simulink model "example_arduino_send_receive"  (R2015b)
settings: Solver=FixedStepAuto  StartTime=0.0  StopTime=1000  FixedStep=1/1000  RelTol=1e-3
libraries: SimFly_System x3
settings Model: ExtModeTrigDuration=2  Creator=marcell  LastModifiedBy=marcell
settings OptimizationCC: OptimizeModelRefInitCode=on  LifeSpan=1  MaxStackSize=64
settings HardwareCC: ProdBitPerPointer=32  ProdLargestAtomicInteger=Long  ProdLargestAtomicFloat=Double  ProdWordSize=32  ProdHWDeviceType=ARM Compatible->ARM Cortex
settings RTWCC: SystemTargetFile=ert.tlc  TemplateMakefile=ert_default_tmf  Description=Embedded Coder  CustomSource=arduino_DUE_wrapper.cpp  Toolchain=Arduino ARM v1.6.1  BuildConfiguration=Faster Runs
settings CodeAppCC: IgnoreCustomStorageClasses=off
settings ERTTargetCC: SupportContinuousTime=on  SupportVariableSizeSignals=on

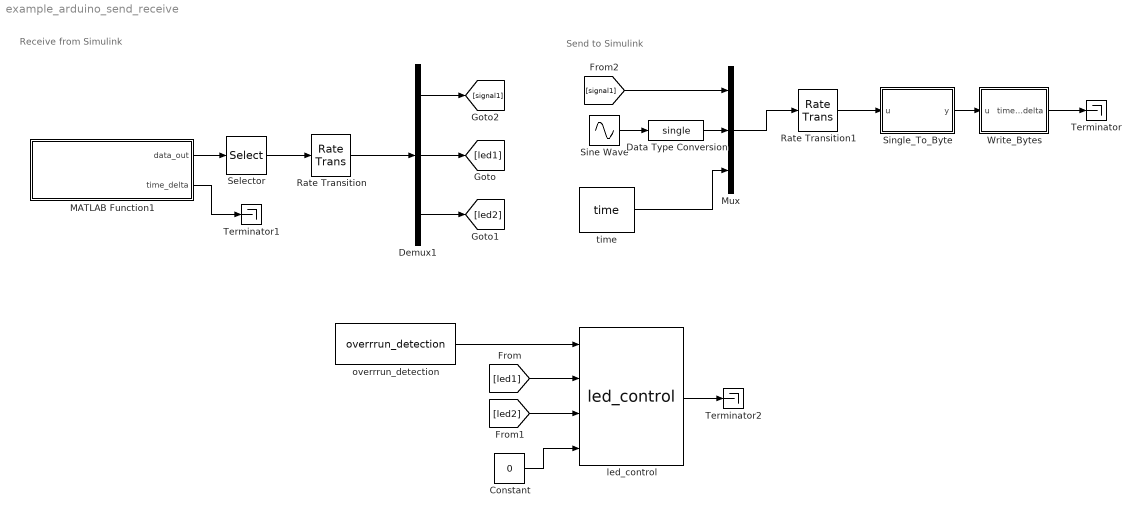
== system example_arduino_send_receive ==
  note: Send to Simulink
  note: Receive from Simulink
  Constant : Constant  Value=0  OutDataTypeStr=boolean
  Data Type Conversion : DataTypeConversion  OutDataTypeStr=single
  Demux1 : Demux  Outputs=3
  MATLAB Function1 : MATLAB Function  TreatAsAtomicUnit=on
  Mux : Mux  Inputs=3
  Rate Transition : RateTransition  OutPortSampleTime=1/1000
  Rate Transition1 : RateTransition  OutPortSampleTime=1/50
  Selector : Selector  InputPortWidth=64  IndexOptions=Index vector (dialog)  Indices=1:3  OutputSizes=1
  Sine Wave : Sin
  Single_To_Byte : MATLAB Function  TreatAsAtomicUnit=on
  Terminator : Terminator
  Terminator1 : Terminator
  Terminator2 : Terminator
  Write_Bytes : MATLAB Function  TreatAsAtomicUnit=on
  led_control : SimFly_System/led_control
  overrrun_detection : SimFly_System/overrrun_detection  sample_time=1/900
  time : SimFly_System/time
  wires:
  overrrun_detection/1 -> led_control/1
  Constant/1 -> led_control/4
  MATLAB Function1/1(data_out) -> Selector/1
  Selector/1 -> Rate Transition/1
  Rate Transition1/1 -> Single_To_Byte/1(u)
  Single_To_Byte/1(y) -> Write_Bytes/1(u)
  Mux/1 -> Rate Transition1/1
  Rate Transition/1 -> Demux1/1
  Write_Bytes/1(time_delta) -> Terminator/1
  MATLAB Function1/2(time_delta) -> Terminator1/1
  led_control/1 -> Terminator2/1
  Demux1/2 -> [led1]
  Demux1/3 -> [led2]
  [led1] -> led_control/2
  [led2] -> led_control/3
  Demux1/1 -> [signal1]
  [signal1] -> Mux/1
  Sine Wave/1 -> Data Type Conversion/1
  time/1 -> Mux/3
  Data Type Conversion/1 -> Mux/2

== matlab function example_arduino_send_receive/MATLAB Function1 ==
  settings: updateMethod=DISCRETE  sampleTime=1/1000
  data: data_out output; time_delta output
function [data_out,time_delta]  = data_receive()
%PURPOSE: (Example) Driver for serial_receive from instrument toolbox
%AUTHOR: Marcell Mocher
%DATE: 3.1.2017
%VERSION: 0.1 V Fist build
%Input: -
%Output: data_out = 
%Info: This drive requires function call triggered simuluink functions in
% order to work
%Requires:  _get_time
%           _serial_init
%           _serial_available
%           _serial_read

persistent init_flag alive_flag state head_count idx data length


data_out = single(zeros(64,1));

if strcmp(coder.target, 'rtw'),
  
time_start = uint32(0);
time_start = coder.ceval('_get_time');

% Parameter from Mask!
baud = uint32(115200); 


% Init parameters

if isempty(init_flag)
    init_flag = 0;
    alive_flag = true;
    length = uint8(1);
    data = uint8(zeros(512,1));
    idx = uint8(1);
    state = uint8(0);
    head_count = uint8(0);
    coder.ceval('_serial_init',uint8(0),baud);   
    coder.ceval('_serial_init',uint8(1),baud);  
end

av = uint8(0);
av = coder.ceval('_serial_available',uint8(0));
if av > 0
    for i = 1:av
        cc = uint8(0);
        cc = coder.ceval('_serial_read',uint8(0));
        switch state
            case 0 %wait for sync 1 (98)
                if cc == 98 
                    state = state + 1;
                    head_count = uint8(1);
                end
            case 1 %wait for sync 1 (98)
                if cc == 98
                    head_count = head_count + 1;
                    if head_count >= 4
                        state = state + 1;
                        idx = uint8(1);
                    end
                else
                    state = uint8(0);
                    head_count = uint8(0);
                end
            case 2 %wait for length
                length = cc;
                state = state + 1;
            case 3 %wait for values
                data(idx) = cc;
                idx = idx + 1;
                if idx > length
                    state = uint8(0);
                end
        end % End of switch (state)
        
    end % End for
    
end % End if

data_out(1:length/4) = typecast(data(1:length),'single');

time_end = uint32(0);
time_end = coder.ceval('_get_time');
time_delta = time_end - time_start;

%coder.ceval('_serial_print',uint8(1),double(data_out(4)));
%coder.ceval('_serial_print',uint8(1),double(0));
else
alive = true;  %TODO: alive flag impementation
time_delta = uint32(0);
end
end

== matlab function example_arduino_send_receive/Write_Bytes ==
  data: u input; time_delta output
function time_delta = write(u)
%PURPOSE: (Example) Driver for Serial writing with hardware abstraction layer
%AUTHOR: Marcell Mocher
%DATE: 3.1.2017
%VERSION: 0.1 V Fist build
%Input: Array to print on the serial port
%Output: Execution time
%Info: This drive requires function call triggered simuluink functions in
% order to work
%Requires:  _get_time
%           _serial_init
%           _serial_print
%           _serial_write
persistent init_flag

if strcmp(coder.target, 'rtw'),
    
    time_start = uint32(0);
    time_start = coder.ceval('_get_time');
    
    if isempty(init_flag)
        init_flag = true;
        coder.ceval('_serial_init',uint8(0),uint32(115200));
    end
    len = uint8(numel(u));
    coder.ceval('_serial_write',uint8(0),u,len);
    
    time_end = uint32(0);
    time_end = coder.ceval('_get_time');
    time_delta = time_end - time_start;
else
    time_delta = uint32(0);
end

== matlab function example_arduino_send_receive/Single_To_Byte ==
  data: u input; y output
function y = SingleToByte(u)
%PURPOSE: (Example) Convertion of single values to a binary array with header and
%terminator
%AUTHOR: Marcell Mocher
%DATE: 3.1.2017
%VERSION: 0.1 V Fist build
%Input: Array of single datatype values
%Output: 

% make sure we're calculating with single 
u = single(u);
% define header %
header = uint8(ones(8,1)*97);
% define terminator %
terminator = uint8([13;10]);

len = numel(u);
% we only have singles%
len_byte = len * 4;
y = uint8(zeros(len_byte+numel(header)+numel(terminator),1));
u_byte = typecast(u,'uint8');
y(1:numel(header)) = header;
for i = 1:numel(u_byte)
   y(i+numel(header)) = u_byte(i) ;
end
y(end-numel(terminator)+1:end) = terminator;
